simulink model "RHex1v3_Z_0v1b"  (Simulink 7.9)
settings: Solver=ode23t  StartTime=0.0  StopTime=tp*3  MaxStep=0.005  RelTol=1e-3
values from neighbouring files (symbols this model uses):
  C = 100    [groundContact_init.m]
  Gvis = 0.01    [groundContact_init.m]
  K = x(5)    [PSO.m]    (also in PSO2_Kconst.m = 865; PSO3_PID.m = 525.4; bClockGen1v3_fin_acc.m = 1000; groundContact_init.m = 1000)
  m = 2    [PSO.m]    (also in PSO2_Kconst.m)
  nux = 1    [groundContact_init.m]
  nuy = 1    [groundContact_init.m]
  psziL = [psziL 360+psziL 720+psziL 1080+psziL]    [bClocGen1v3_fun.m]    (also in bClockGen1v3_fin_acc.m)
  psziR = [psziR 360+psziR 720+psziR 1080+psziR]    [bClocGen1v3_fun.m]    (also in bClockGen1v3_fin_acc.m)
  tp = x(1)    [PSO.m]    (also in PSO2_Kconst.m; PSO3_PID.m = 1.6; bClockGen1v3_fin_acc.m = 3)
undefined symbols (not defined in the file or in its folder): Body, deg, lab_rogz1v1, RHex1v3, RHex1v3_Z, RootPart, s
libraries: mblibv1 x61, Ervin x12, simulink x8
(part 2 of 2)

== system RHex1v3_Z_0v1b/Left_Middle/TorqueControl ==
  note: TauControl
  ref : Inport
  sensor : Inport  Port=2
  Continuous Angle : mblibv1/Utilities/Continuous Angle  rad=deg  rads=deg/s
  Demux2 : Demux
  Gain2 : Gain  Gain=Gvis
  PID : simulink/Continuous/PID Controller  Controller=PID  TimeDomain=Continuous-time  SampleTime=1  IntegratorMethod=Forward Euler  FilterMethod=Forward Euler  Form=Parallel  P=100  I=2  D=10  N=0.00001  InitialConditionSource=internal  InitialConditionForIntegrator=0  InitialConditionForFilter=0  ExternalReset=none  LimitOutput=off  UpperSaturationLimit=inf  LowerSaturationLimit=-inf  LinearizeAsGain=off  AntiWindupMode=none  Kb=1  TrackingMode=off  Kt=1  PParamMin=[]  PParamMax=[]  IParamMin=[]  IParamMax=[]  DParamMin=[]  DParamMax=[]  NParamMin=[]  NParamMax=[]  KbParamMin=[]  KbParamMax=[]  KtParamMin=[]  KtParamMax=[]  POutMin=[]  POutMax=[]  IOutMin=[]  IOutMax=[]  DOutMin=[]  DOutMax=[]  NOutMin=[]  NOutMax=[]  KbOutMin=[]  KbOutMax=[]  KtOutMin=[]  KtOutMax=[]  IntegratorOutMin=[]  IntegratorOutMax=[]  FilterOutMin=[]  FilterOutMax=[]  SumOutMin=[]  SumOutMax=[]  SumI1OutMin=[]  SumI1OutMax=[]  SumI2OutMin=[]  SumI2OutMax=[]  SumI3OutMin=[]  SumI3OutMax=[]  SumDOutMin=[]  SumDOutMax=[]  SaturationOutMin=[]  SaturationOutMax=[]  IntegratorContinuousStateAttributes=''  IntegratorStateMustResolveToSignalObject=off  IntegratorRTWStateStorageClass=Auto  FilterContinuousStateAttributes=''  FilterStateMustResolveToSignalObject=off  FilterRTWStateStorageClass=Auto
  Sum1 : Sum  Inputs=|+-
  Sum2 : Sum  Inputs=|+-
  u : Outport
  wires:
  Demux2/1 -> Continuous Angle/1  "theta"
  sensor/1 -> Demux2/1
  PID/1 -> Sum2/1
  Sum2/1 -> u/1
  ref/1 -> Sum1/1  "referent_signal"
  Demux2/2 -> Gain2/1, Continuous Angle/2  "dtheta"
  Continuous Angle/1 -> Sum1/2
  Sum1/1 -> PID/1  "error"
  Gain2/1 -> Sum2/2  "viscous_damping"

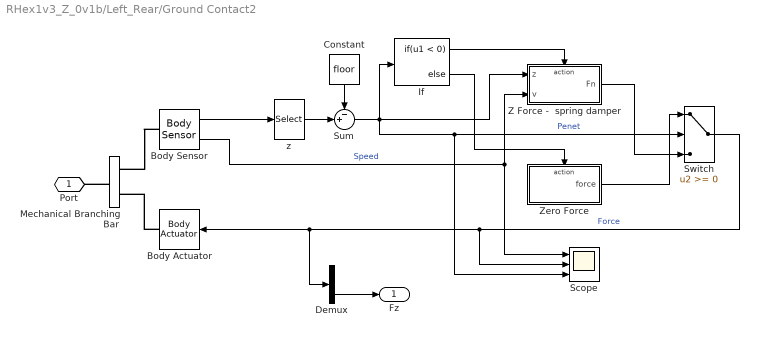
== system RHex1v3_Z_0v1b/Left_Rear/Ground Contact2 ==
  Body Actuator : mblibv1/Sensors &  Actuators/Body Actuator  UpdateFromCAD=off  PhysicalDomain=Mechanical  PortType=blob  ActuationStyle=Force  AngleUnits=deg  ArcVelocityUnits=deg/s  ArcAccelerationUnits=deg/s^2  CoordPositionUnits=m  VelocityUnits=m/s  AccelerationUnits=m/s^2  ForceUnits=N  TorqueUnits=N*m  ActiveIO=on  Width=3  DialogClass=MechanicalActuatorBlock  ReferenceFrame=Absolute (World)  Angle=off  CoordPosition=on  Force=on  Torque=off
  Body Sensor : mblibv1/Sensors &  Actuators/Body Sensor  UpdateFromCAD=off  PhysicalDomain=Mechanical  PortType=blob  Muxed=off  Pose=off  Angle=on  AngleUnits=deg  ArcVelocity=off  ArcVelocityUnits=deg/s  ArcAcceleration=off  ArcAccelerationUnits=deg/s^2  CoordPosition=on  CoordPositionUnits=m  Velocity=on  VelocityUnits=m/s  Acceleration=off  AccelerationUnits=m/s^2  Quaternion=on  QuaternionDT=off  QuaternionDDT=off  QuaternionUnits=off  OutputVector=[ 3 3 ]  ActiveIO=on  Width=6  DialogClass=MechanicalSensorBlock  ReferenceFrame=Absolute (World)
  Constant : Constant  Value=floor
  Demux : Demux  Outputs=3
  If : If  IfExpression=u1 < 0
  Mechanical Branching Bar : mblibv1/Utilities/Mechanical Branching Bar  LConnTagsString=_newl0  RConnTagsString=SA0|SA1  UpdateFromCAD=off  DialogClass=MechanicalBranchingBarBlock  NumSAPorts=2
  Scope : Scope  NumInputPorts=3
      settings: YMin=-0.11~-15~-0.025  YMax=0.02~27.5~0.015
  Sum : Sum  Inputs=-+|  SaturateOnIntegerOverflow=on
  Switch : Switch
  Z Force -  spring damper : Subsystem  TreatAsAtomicUnit=on  mask{K=K, C=C, nux=nux, nuy=nuy}
  Zero Force : Subsystem  TreatAsAtomicUnit=on
  z : Selector  InputPortWidth=3  IndexOptions=Index vector (dialog)  Indices=[3]  OutputSizes=1
  Port : PMIOPort  Port=1  Side=Left
  Fz : Outport
  wires:
  Z Force -  spring damper/1(Fn) -> Switch/3
  Zero Force/1(force) -> Switch/1
  Constant/1 -> Sum/1
  Sum/1 -> Switch/2, Scope/3, Z Force -  spring damper/1(z), If/1  "Penet"
  z/1 -> Sum/2
  Switch/1 -> Scope/2, Body Actuator/1, Demux/1  "Force"
  If/1 -> Z Force -  spring damper/Action
  If/2 -> Zero Force/Action
  Body Sensor/2 -> Scope/1, Z Force -  spring damper/2(v)  "Speed"
  Body Sensor/1 -> z/1
  Demux/3 -> Fz/1
  connections:
  Mechanical Branching Bar/LConn1 -- Port/RConn1
  Body Actuator/RConn1 -- Mechanical Branching Bar/RConn2
  Body Sensor/LConn1 -- Mechanical Branching Bar/RConn1

== system RHex1v3_Z_0v1b/Left_Rear/TorqueControl ==
  note: TauControl
  ref : Inport
  sensor : Inport  Port=2
  Continuous Angle : mblibv1/Utilities/Continuous Angle  rad=deg  rads=deg/s
  Demux2 : Demux
  Gain2 : Gain  Gain=Gvis
  PID : simulink/Continuous/PID Controller  Controller=PID  TimeDomain=Continuous-time  SampleTime=1  IntegratorMethod=Forward Euler  FilterMethod=Forward Euler  Form=Parallel  P=100  I=2  D=10  N=0.00001  InitialConditionSource=internal  InitialConditionForIntegrator=0  InitialConditionForFilter=0  ExternalReset=none  LimitOutput=off  UpperSaturationLimit=inf  LowerSaturationLimit=-inf  LinearizeAsGain=off  AntiWindupMode=none  Kb=1  TrackingMode=off  Kt=1  PParamMin=[]  PParamMax=[]  IParamMin=[]  IParamMax=[]  DParamMin=[]  DParamMax=[]  NParamMin=[]  NParamMax=[]  KbParamMin=[]  KbParamMax=[]  KtParamMin=[]  KtParamMax=[]  POutMin=[]  POutMax=[]  IOutMin=[]  IOutMax=[]  DOutMin=[]  DOutMax=[]  NOutMin=[]  NOutMax=[]  KbOutMin=[]  KbOutMax=[]  KtOutMin=[]  KtOutMax=[]  IntegratorOutMin=[]  IntegratorOutMax=[]  FilterOutMin=[]  FilterOutMax=[]  SumOutMin=[]  SumOutMax=[]  SumI1OutMin=[]  SumI1OutMax=[]  SumI2OutMin=[]  SumI2OutMax=[]  SumI3OutMin=[]  SumI3OutMax=[]  SumDOutMin=[]  SumDOutMax=[]  SaturationOutMin=[]  SaturationOutMax=[]  IntegratorContinuousStateAttributes=''  IntegratorStateMustResolveToSignalObject=off  IntegratorRTWStateStorageClass=Auto  FilterContinuousStateAttributes=''  FilterStateMustResolveToSignalObject=off  FilterRTWStateStorageClass=Auto
  Sum1 : Sum  Inputs=|+-
  Sum2 : Sum  Inputs=|+-
  u : Outport
  wires:
  Demux2/1 -> Continuous Angle/1  "theta"
  sensor/1 -> Demux2/1
  PID/1 -> Sum2/1
  Sum2/1 -> u/1
  ref/1 -> Sum1/1  "referent_signal"
  Demux2/2 -> Gain2/1, Continuous Angle/2  "dtheta"
  Continuous Angle/1 -> Sum1/2
  Sum1/1 -> PID/1  "error"
  Gain2/1 -> Sum2/2  "viscous_damping"

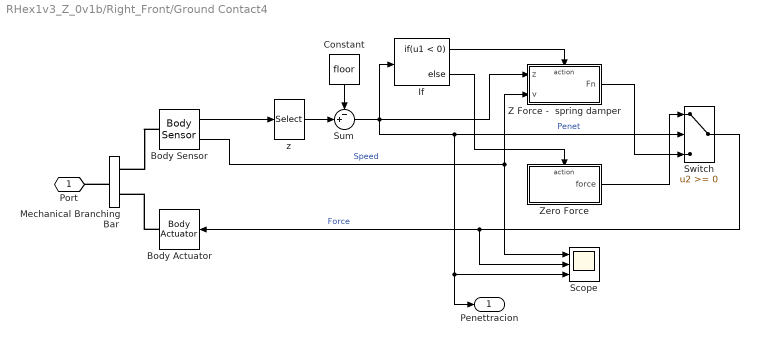
== system RHex1v3_Z_0v1b/Right_Front/Ground Contact4 ==
  Body Actuator : mblibv1/Sensors &  Actuators/Body Actuator  UpdateFromCAD=off  PhysicalDomain=Mechanical  PortType=blob  ActuationStyle=Force  AngleUnits=deg  ArcVelocityUnits=deg/s  ArcAccelerationUnits=deg/s^2  CoordPositionUnits=m  VelocityUnits=m/s  AccelerationUnits=m/s^2  ForceUnits=N  TorqueUnits=N*m  ActiveIO=on  Width=3  DialogClass=MechanicalActuatorBlock  ReferenceFrame=Absolute (World)  Angle=off  CoordPosition=on  Force=on  Torque=off
  Body Sensor : mblibv1/Sensors &  Actuators/Body Sensor  UpdateFromCAD=off  PhysicalDomain=Mechanical  PortType=blob  Muxed=off  Pose=off  Angle=on  AngleUnits=deg  ArcVelocity=off  ArcVelocityUnits=deg/s  ArcAcceleration=off  ArcAccelerationUnits=deg/s^2  CoordPosition=on  CoordPositionUnits=m  Velocity=on  VelocityUnits=m/s  Acceleration=off  AccelerationUnits=m/s^2  Quaternion=on  QuaternionDT=off  QuaternionDDT=off  QuaternionUnits=off  OutputVector=[ 3 3 ]  ActiveIO=on  Width=6  DialogClass=MechanicalSensorBlock  ReferenceFrame=Absolute (World)
  Constant : Constant  Value=floor
  If : If  IfExpression=u1 < 0
  Mechanical Branching Bar : mblibv1/Utilities/Mechanical Branching Bar  LConnTagsString=_newl0  RConnTagsString=SA0|SA1  UpdateFromCAD=off  DialogClass=MechanicalBranchingBarBlock  NumSAPorts=2
  Scope : Scope  NumInputPorts=3
      settings: YMin=-0.11~-15~-0.025  YMax=0.02~27.5~0.015
  Sum : Sum  Inputs=-+|  SaturateOnIntegerOverflow=on
  Switch : Switch
  Z Force -  spring damper : Subsystem  TreatAsAtomicUnit=on  mask{K=K, C=C, nux=nux, nuy=nuy}
  Zero Force : Subsystem  TreatAsAtomicUnit=on
  z : Selector  InputPortWidth=3  IndexOptions=Index vector (dialog)  Indices=[3]  OutputSizes=1
  Port : PMIOPort  Port=1  Side=Left
  Penettracion : Outport
  wires:
  Body Sensor/1 -> z/1
  Body Sensor/2 -> Z Force -  spring damper/2(v), Scope/1  "Speed"
  If/2 -> Zero Force/Action
  If/1 -> Z Force -  spring damper/Action
  Switch/1 -> Body Actuator/1, Scope/2  "Force"
  z/1 -> Sum/2
  Sum/1 -> If/1, Z Force -  spring damper/1(z), Penettracion/1, Scope/3, Switch/2  "Penet"
  Constant/1 -> Sum/1
  Zero Force/1(force) -> Switch/1
  Z Force -  spring damper/1(Fn) -> Switch/3
  connections:
  Body Sensor/LConn1 -- Mechanical Branching Bar/RConn1
  Body Actuator/RConn1 -- Mechanical Branching Bar/RConn2
  Mechanical Branching Bar/LConn1 -- Port/RConn1

== system RHex1v3_Z_0v1b/Right_Front/TorqueControl1 ==
  note: TauControl
  ref : Inport
  sensor : Inport  Port=2
  Continuous Angle : mblibv1/Utilities/Continuous Angle  rad=deg  rads=deg/s
  Demux2 : Demux
  Gain2 : Gain  Gain=Gvis
  PID : simulink/Continuous/PID Controller  Controller=PID  TimeDomain=Continuous-time  SampleTime=1  IntegratorMethod=Forward Euler  FilterMethod=Forward Euler  Form=Parallel  P=100  I=2  D=10  N=0.00001  InitialConditionSource=internal  InitialConditionForIntegrator=0  InitialConditionForFilter=0  ExternalReset=none  LimitOutput=off  UpperSaturationLimit=inf  LowerSaturationLimit=-inf  LinearizeAsGain=off  AntiWindupMode=none  Kb=1  TrackingMode=off  Kt=1  PParamMin=[]  PParamMax=[]  IParamMin=[]  IParamMax=[]  DParamMin=[]  DParamMax=[]  NParamMin=[]  NParamMax=[]  KbParamMin=[]  KbParamMax=[]  KtParamMin=[]  KtParamMax=[]  POutMin=[]  POutMax=[]  IOutMin=[]  IOutMax=[]  DOutMin=[]  DOutMax=[]  NOutMin=[]  NOutMax=[]  KbOutMin=[]  KbOutMax=[]  KtOutMin=[]  KtOutMax=[]  IntegratorOutMin=[]  IntegratorOutMax=[]  FilterOutMin=[]  FilterOutMax=[]  SumOutMin=[]  SumOutMax=[]  SumI1OutMin=[]  SumI1OutMax=[]  SumI2OutMin=[]  SumI2OutMax=[]  SumI3OutMin=[]  SumI3OutMax=[]  SumDOutMin=[]  SumDOutMax=[]  SaturationOutMin=[]  SaturationOutMax=[]  IntegratorContinuousStateAttributes=''  IntegratorStateMustResolveToSignalObject=off  IntegratorRTWStateStorageClass=Auto  FilterContinuousStateAttributes=''  FilterStateMustResolveToSignalObject=off  FilterRTWStateStorageClass=Auto
  Sum1 : Sum  Inputs=|+-
  Sum2 : Sum  Inputs=|+-
  u : Outport
  wires:
  Gain2/1 -> Sum2/2  "viscous_damping"
  Sum1/1 -> PID/1  "error"
  Continuous Angle/1 -> Sum1/2
  Demux2/2 -> Continuous Angle/2, Gain2/1  "dtheta"
  ref/1 -> Sum1/1  "referent_signal"
  Sum2/1 -> u/1
  PID/1 -> Sum2/1
  sensor/1 -> Demux2/1
  Demux2/1 -> Continuous Angle/1  "theta"

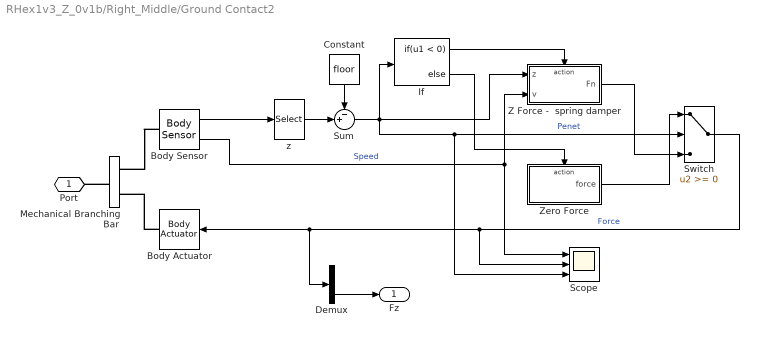
== system RHex1v3_Z_0v1b/Right_Middle/Ground Contact2 ==
  Body Actuator : mblibv1/Sensors &  Actuators/Body Actuator  UpdateFromCAD=off  PhysicalDomain=Mechanical  PortType=blob  ActuationStyle=Force  AngleUnits=deg  ArcVelocityUnits=deg/s  ArcAccelerationUnits=deg/s^2  CoordPositionUnits=m  VelocityUnits=m/s  AccelerationUnits=m/s^2  ForceUnits=N  TorqueUnits=N*m  ActiveIO=on  Width=3  DialogClass=MechanicalActuatorBlock  ReferenceFrame=Absolute (World)  Angle=off  CoordPosition=on  Force=on  Torque=off
  Body Sensor : mblibv1/Sensors &  Actuators/Body Sensor  UpdateFromCAD=off  PhysicalDomain=Mechanical  PortType=blob  Muxed=off  Pose=off  Angle=on  AngleUnits=deg  ArcVelocity=off  ArcVelocityUnits=deg/s  ArcAcceleration=off  ArcAccelerationUnits=deg/s^2  CoordPosition=on  CoordPositionUnits=m  Velocity=on  VelocityUnits=m/s  Acceleration=off  AccelerationUnits=m/s^2  Quaternion=on  QuaternionDT=off  QuaternionDDT=off  QuaternionUnits=off  OutputVector=[ 3 3 ]  ActiveIO=on  Width=6  DialogClass=MechanicalSensorBlock  ReferenceFrame=Absolute (World)
  Constant : Constant  Value=floor
  Demux : Demux  Outputs=3
  If : If  IfExpression=u1 < 0
  Mechanical Branching Bar : mblibv1/Utilities/Mechanical Branching Bar  LConnTagsString=_newl0  RConnTagsString=SA0|SA1  UpdateFromCAD=off  DialogClass=MechanicalBranchingBarBlock  NumSAPorts=2
  Scope : Scope  NumInputPorts=3
      settings: YMin=-0.11~-15~-0.025  YMax=0.02~27.5~0.015
  Sum : Sum  Inputs=-+|  SaturateOnIntegerOverflow=on
  Switch : Switch
  Z Force -  spring damper : Subsystem  TreatAsAtomicUnit=on  mask{K=K, C=C, nux=nux, nuy=nuy}
  Zero Force : Subsystem  TreatAsAtomicUnit=on
  z : Selector  InputPortWidth=3  IndexOptions=Index vector (dialog)  Indices=[3]  OutputSizes=1
  Port : PMIOPort  Port=1  Side=Left
  Fz : Outport
  wires:
  Z Force -  spring damper/1(Fn) -> Switch/3
  Zero Force/1(force) -> Switch/1
  Constant/1 -> Sum/1
  Sum/1 -> Switch/2, Scope/3, Z Force -  spring damper/1(z), If/1  "Penet"
  z/1 -> Sum/2
  Switch/1 -> Scope/2, Body Actuator/1, Demux/1  "Force"
  If/1 -> Z Force -  spring damper/Action
  If/2 -> Zero Force/Action
  Body Sensor/2 -> Scope/1, Z Force -  spring damper/2(v)  "Speed"
  Body Sensor/1 -> z/1
  Demux/3 -> Fz/1
  connections:
  Mechanical Branching Bar/LConn1 -- Port/RConn1
  Body Actuator/RConn1 -- Mechanical Branching Bar/RConn2
  Body Sensor/LConn1 -- Mechanical Branching Bar/RConn1

== system RHex1v3_Z_0v1b/Right_Middle/TorqueControl1 ==
  note: TauControl
  ref : Inport
  sensor : Inport  Port=2
  Continuous Angle : mblibv1/Utilities/Continuous Angle  rad=deg  rads=deg/s
  Demux2 : Demux
  Gain2 : Gain  Gain=Gvis
  PID : simulink/Continuous/PID Controller  Controller=PID  TimeDomain=Continuous-time  SampleTime=1  IntegratorMethod=Forward Euler  FilterMethod=Forward Euler  Form=Parallel  P=100  I=2  D=10  N=0.00001  InitialConditionSource=internal  InitialConditionForIntegrator=0  InitialConditionForFilter=0  ExternalReset=none  LimitOutput=off  UpperSaturationLimit=inf  LowerSaturationLimit=-inf  LinearizeAsGain=off  AntiWindupMode=none  Kb=1  TrackingMode=off  Kt=1  PParamMin=[]  PParamMax=[]  IParamMin=[]  IParamMax=[]  DParamMin=[]  DParamMax=[]  NParamMin=[]  NParamMax=[]  KbParamMin=[]  KbParamMax=[]  KtParamMin=[]  KtParamMax=[]  POutMin=[]  POutMax=[]  IOutMin=[]  IOutMax=[]  DOutMin=[]  DOutMax=[]  NOutMin=[]  NOutMax=[]  KbOutMin=[]  KbOutMax=[]  KtOutMin=[]  KtOutMax=[]  IntegratorOutMin=[]  IntegratorOutMax=[]  FilterOutMin=[]  FilterOutMax=[]  SumOutMin=[]  SumOutMax=[]  SumI1OutMin=[]  SumI1OutMax=[]  SumI2OutMin=[]  SumI2OutMax=[]  SumI3OutMin=[]  SumI3OutMax=[]  SumDOutMin=[]  SumDOutMax=[]  SaturationOutMin=[]  SaturationOutMax=[]  IntegratorContinuousStateAttributes=''  IntegratorStateMustResolveToSignalObject=off  IntegratorRTWStateStorageClass=Auto  FilterContinuousStateAttributes=''  FilterStateMustResolveToSignalObject=off  FilterRTWStateStorageClass=Auto
  Sum1 : Sum  Inputs=|+-
  Sum2 : Sum  Inputs=|+-
  u : Outport
  wires:
  Gain2/1 -> Sum2/2  "viscous_damping"
  Sum1/1 -> PID/1  "error"
  Continuous Angle/1 -> Sum1/2
  Demux2/2 -> Continuous Angle/2, Gain2/1  "dtheta"
  ref/1 -> Sum1/1  "referent_signal"
  Sum2/1 -> u/1
  PID/1 -> Sum2/1
  sensor/1 -> Demux2/1
  Demux2/1 -> Continuous Angle/1  "theta"

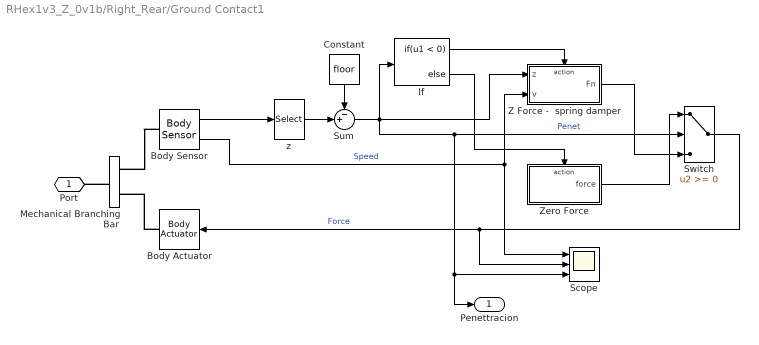
== system RHex1v3_Z_0v1b/Right_Rear/Ground Contact1 ==
  Body Actuator : mblibv1/Sensors &  Actuators/Body Actuator  UpdateFromCAD=off  PhysicalDomain=Mechanical  PortType=blob  ActuationStyle=Force  AngleUnits=deg  ArcVelocityUnits=deg/s  ArcAccelerationUnits=deg/s^2  CoordPositionUnits=m  VelocityUnits=m/s  AccelerationUnits=m/s^2  ForceUnits=N  TorqueUnits=N*m  ActiveIO=on  Width=3  DialogClass=MechanicalActuatorBlock  ReferenceFrame=Absolute (World)  Angle=off  CoordPosition=on  Force=on  Torque=off
  Body Sensor : mblibv1/Sensors &  Actuators/Body Sensor  UpdateFromCAD=off  PhysicalDomain=Mechanical  PortType=blob  Muxed=off  Pose=off  Angle=on  AngleUnits=deg  ArcVelocity=off  ArcVelocityUnits=deg/s  ArcAcceleration=off  ArcAccelerationUnits=deg/s^2  CoordPosition=on  CoordPositionUnits=m  Velocity=on  VelocityUnits=m/s  Acceleration=off  AccelerationUnits=m/s^2  Quaternion=on  QuaternionDT=off  QuaternionDDT=off  QuaternionUnits=off  OutputVector=[ 3 3 ]  ActiveIO=on  Width=6  DialogClass=MechanicalSensorBlock  ReferenceFrame=Absolute (World)
  Constant : Constant  Value=floor
  If : If  IfExpression=u1 < 0
  Mechanical Branching Bar : mblibv1/Utilities/Mechanical Branching Bar  LConnTagsString=_newl0  RConnTagsString=SA0|SA1  UpdateFromCAD=off  DialogClass=MechanicalBranchingBarBlock  NumSAPorts=2
  Scope : Scope  NumInputPorts=3
      settings: YMin=-0.11~-15~-0.025  YMax=0.02~27.5~0.015
  Sum : Sum  Inputs=-+|  SaturateOnIntegerOverflow=on
  Switch : Switch
  Z Force -  spring damper : Subsystem  TreatAsAtomicUnit=on  mask{K=K, C=C, nux=nux, nuy=nuy}
  Zero Force : Subsystem  TreatAsAtomicUnit=on
  z : Selector  InputPortWidth=3  IndexOptions=Index vector (dialog)  Indices=[3]  OutputSizes=1
  Port : PMIOPort  Port=1  Side=Left
  Penettracion : Outport
  wires:
  Body Sensor/1 -> z/1
  Body Sensor/2 -> Z Force -  spring damper/2(v), Scope/1  "Speed"
  If/2 -> Zero Force/Action
  If/1 -> Z Force -  spring damper/Action
  Switch/1 -> Body Actuator/1, Scope/2  "Force"
  z/1 -> Sum/2
  Sum/1 -> If/1, Z Force -  spring damper/1(z), Penettracion/1, Scope/3, Switch/2  "Penet"
  Constant/1 -> Sum/1
  Zero Force/1(force) -> Switch/1
  Z Force -  spring damper/1(Fn) -> Switch/3
  connections:
  Body Sensor/LConn1 -- Mechanical Branching Bar/RConn1
  Body Actuator/RConn1 -- Mechanical Branching Bar/RConn2
  Mechanical Branching Bar/LConn1 -- Port/RConn1

== system RHex1v3_Z_0v1b/Right_Rear/TorqueControl ==
  note: TauControl
  ref : Inport
  sensor : Inport  Port=2
  Continuous Angle : mblibv1/Utilities/Continuous Angle  rad=deg  rads=deg/s
  Demux2 : Demux
  Gain2 : Gain  Gain=Gvis
  PID : simulink/Continuous/PID Controller  Controller=PID  TimeDomain=Continuous-time  SampleTime=1  IntegratorMethod=Forward Euler  FilterMethod=Forward Euler  Form=Parallel  P=100  I=2  D=10  N=0.00001  InitialConditionSource=internal  InitialConditionForIntegrator=0  InitialConditionForFilter=0  ExternalReset=none  LimitOutput=off  UpperSaturationLimit=inf  LowerSaturationLimit=-inf  LinearizeAsGain=off  AntiWindupMode=none  Kb=1  TrackingMode=off  Kt=1  PParamMin=[]  PParamMax=[]  IParamMin=[]  IParamMax=[]  DParamMin=[]  DParamMax=[]  NParamMin=[]  NParamMax=[]  KbParamMin=[]  KbParamMax=[]  KtParamMin=[]  KtParamMax=[]  POutMin=[]  POutMax=[]  IOutMin=[]  IOutMax=[]  DOutMin=[]  DOutMax=[]  NOutMin=[]  NOutMax=[]  KbOutMin=[]  KbOutMax=[]  KtOutMin=[]  KtOutMax=[]  IntegratorOutMin=[]  IntegratorOutMax=[]  FilterOutMin=[]  FilterOutMax=[]  SumOutMin=[]  SumOutMax=[]  SumI1OutMin=[]  SumI1OutMax=[]  SumI2OutMin=[]  SumI2OutMax=[]  SumI3OutMin=[]  SumI3OutMax=[]  SumDOutMin=[]  SumDOutMax=[]  SaturationOutMin=[]  SaturationOutMax=[]  IntegratorContinuousStateAttributes=''  IntegratorStateMustResolveToSignalObject=off  IntegratorRTWStateStorageClass=Auto  FilterContinuousStateAttributes=''  FilterStateMustResolveToSignalObject=off  FilterRTWStateStorageClass=Auto
  Sum1 : Sum  Inputs=|+-
  Sum2 : Sum  Inputs=|+-
  u : Outport
  wires:
  Demux2/1 -> Continuous Angle/1  "theta"
  sensor/1 -> Demux2/1
  PID/1 -> Sum2/1
  Sum2/1 -> u/1
  ref/1 -> Sum1/1  "referent_signal"
  Demux2/2 -> Gain2/1, Continuous Angle/2  "dtheta"
  Continuous Angle/1 -> Sum1/2
  Sum1/1 -> PID/1  "error"
  Gain2/1 -> Sum2/2  "viscous_damping"

== system RHex1v3_Z_0v1b/Left_Front/Ground Contact2/Z Force -  spring damper ==
  z : Inport
  v : Inport  Port=2
  Action Port : ActionPort  ActionType=then
  Add : Sum  Inputs=--
  Demux : Demux  Outputs=3
  Gain : Gain  Gain=K
  Gain1 : Gain  Gain=C
  Mux : Mux  Inputs=3
  Simple friction X : Ervin/Simple friction  nu=nux
  Simple friction Y : Ervin/Simple friction  nu=nuy
  Fn : Outport  InitialOutput=0
  wires:
  Simple friction X/1 -> Mux/1
  Simple friction Y/1 -> Mux/2
  Demux/1 -> Simple friction X/1
  z/1 -> Gain/1
  Gain1/1 -> Add/1
  Mux/1 -> Fn/1
  Demux/2 -> Simple friction Y/1
  Demux/3 -> Gain1/1
  v/1 -> Demux/1
  Gain/1 -> Add/2
  Add/1 -> Mux/3, Simple friction X/2, Simple friction Y/2

== system RHex1v3_Z_0v1b/Left_Front/Ground Contact2/Zero Force ==
  Action Port : ActionPort  ActionType=else
  Zero Force : Constant  Value=[0 0 0]
  force : Outport  InitialOutput=0
  wires:
  Zero Force/1 -> force/1

== system RHex1v3_Z_0v1b/Left_Middle/Ground Contact6/Z Force -  spring damper ==
  z : Inport
  v : Inport  Port=2
  Action Port : ActionPort  ActionType=then
  Add : Sum  Inputs=--
  Demux : Demux  Outputs=3
  Gain : Gain  Gain=K
  Gain1 : Gain  Gain=C
  Mux : Mux  Inputs=3
  Simple friction X : Ervin/Simple friction  nu=nux
  Simple friction Y : Ervin/Simple friction  nu=nuy
  Fn : Outport  InitialOutput=0
  wires:
  Simple friction X/1 -> Mux/1
  Simple friction Y/1 -> Mux/2
  Demux/1 -> Simple friction X/1
  z/1 -> Gain/1
  Gain1/1 -> Add/1
  Mux/1 -> Fn/1
  Demux/2 -> Simple friction Y/1
  Demux/3 -> Gain1/1
  v/1 -> Demux/1
  Gain/1 -> Add/2
  Add/1 -> Mux/3, Simple friction X/2, Simple friction Y/2

== system RHex1v3_Z_0v1b/Left_Middle/Ground Contact6/Zero Force ==
  Action Port : ActionPort  ActionType=else
  Zero Force : Constant  Value=[0 0 0]
  force : Outport  InitialOutput=0
  wires:
  Zero Force/1 -> force/1

== system RHex1v3_Z_0v1b/Left_Rear/Ground Contact2/Z Force -  spring damper ==
  z : Inport
  v : Inport  Port=2
  Action Port : ActionPort  ActionType=then
  Add : Sum  Inputs=--
  Demux : Demux  Outputs=3
  Gain : Gain  Gain=K
  Gain1 : Gain  Gain=C
  Mux : Mux  Inputs=3
  Simple friction X : Ervin/Simple friction  nu=nux
  Simple friction Y : Ervin/Simple friction  nu=nuy
  Fn : Outport  InitialOutput=0
  wires:
  Simple friction X/1 -> Mux/1
  Simple friction Y/1 -> Mux/2
  Demux/1 -> Simple friction X/1
  z/1 -> Gain/1
  Gain1/1 -> Add/1
  Mux/1 -> Fn/1
  Demux/2 -> Simple friction Y/1
  Demux/3 -> Gain1/1
  v/1 -> Demux/1
  Gain/1 -> Add/2
  Add/1 -> Mux/3, Simple friction X/2, Simple friction Y/2

== system RHex1v3_Z_0v1b/Left_Rear/Ground Contact2/Zero Force ==
  Action Port : ActionPort  ActionType=else
  Zero Force : Constant  Value=[0 0 0]
  force : Outport  InitialOutput=0
  wires:
  Zero Force/1 -> force/1

== system RHex1v3_Z_0v1b/Right_Front/Ground Contact4/Z Force -  spring damper ==
  z : Inport
  v : Inport  Port=2
  Action Port : ActionPort  ActionType=then
  Add : Sum  Inputs=--
  Demux : Demux  Outputs=3
  Gain : Gain  Gain=K
  Gain1 : Gain  Gain=C
  Mux : Mux  Inputs=3
  Simple friction X : Ervin/Simple friction  nu=nux
  Simple friction Y : Ervin/Simple friction  nu=nuy
  Fn : Outport  InitialOutput=0
  wires:
  Add/1 -> Simple friction Y/2, Simple friction X/2, Mux/3
  Gain/1 -> Add/2
  v/1 -> Demux/1
  Demux/3 -> Gain1/1
  Demux/2 -> Simple friction Y/1
  Mux/1 -> Fn/1
  Gain1/1 -> Add/1
  z/1 -> Gain/1
  Demux/1 -> Simple friction X/1
  Simple friction Y/1 -> Mux/2
  Simple friction X/1 -> Mux/1

== system RHex1v3_Z_0v1b/Right_Front/Ground Contact4/Zero Force ==
  Action Port : ActionPort  ActionType=else
  Zero Force : Constant  Value=[0 0 0]
  force : Outport  InitialOutput=0
  wires:
  Zero Force/1 -> force/1

== system RHex1v3_Z_0v1b/Right_Middle/Ground Contact2/Z Force -  spring damper ==
  z : Inport
  v : Inport  Port=2
  Action Port : ActionPort  ActionType=then
  Add : Sum  Inputs=--
  Demux : Demux  Outputs=3
  Gain : Gain  Gain=K
  Gain1 : Gain  Gain=C
  Mux : Mux  Inputs=3
  Simple friction X : Ervin/Simple friction  nu=nux
  Simple friction Y : Ervin/Simple friction  nu=nuy
  Fn : Outport  InitialOutput=0
  wires:
  Simple friction X/1 -> Mux/1
  Simple friction Y/1 -> Mux/2
  Demux/1 -> Simple friction X/1
  z/1 -> Gain/1
  Gain1/1 -> Add/1
  Mux/1 -> Fn/1
  Demux/2 -> Simple friction Y/1
  Demux/3 -> Gain1/1
  v/1 -> Demux/1
  Gain/1 -> Add/2
  Add/1 -> Mux/3, Simple friction X/2, Simple friction Y/2

== system RHex1v3_Z_0v1b/Right_Middle/Ground Contact2/Zero Force ==
  Action Port : ActionPort  ActionType=else
  Zero Force : Constant  Value=[0 0 0]
  force : Outport  InitialOutput=0
  wires:
  Zero Force/1 -> force/1

== system RHex1v3_Z_0v1b/Right_Rear/Ground Contact1/Z Force -  spring damper ==
  z : Inport
  v : Inport  Port=2
  Action Port : ActionPort  ActionType=then
  Add : Sum  Inputs=--
  Demux : Demux  Outputs=3
  Gain : Gain  Gain=K
  Gain1 : Gain  Gain=C
  Mux : Mux  Inputs=3
  Simple friction X : Ervin/Simple friction  nu=nux
  Simple friction Y : Ervin/Simple friction  nu=nuy
  Fn : Outport  InitialOutput=0
  wires:
  Add/1 -> Simple friction Y/2, Simple friction X/2, Mux/3
  Gain/1 -> Add/2
  v/1 -> Demux/1
  Demux/3 -> Gain1/1
  Demux/2 -> Simple friction Y/1
  Mux/1 -> Fn/1
  Gain1/1 -> Add/1
  z/1 -> Gain/1
  Demux/1 -> Simple friction X/1
  Simple friction Y/1 -> Mux/2
  Simple friction X/1 -> Mux/1

== system RHex1v3_Z_0v1b/Right_Rear/Ground Contact1/Zero Force ==
  Action Port : ActionPort  ActionType=else
  Zero Force : Constant  Value=[0 0 0]
  force : Outport  InitialOutput=0
  wires:
  Zero Force/1 -> force/1
